simulink model "new_lv_try_control2"  (Simulink 7.1)
settings: Solver=ode3  StartTime=0.0  StopTime=150  FixedStep=0.01  RelTol=1e-3
values from neighbouring files (symbols this model uses):
  C = abs(d-B)    [fuzzycontrol.m]    (also in lv_demofile6.m = 1450000)
  Jem = 90    [lv_cankaofile.m]    (also in lv_demofile.m = 97.5; lv_demofile1.m = 97.5; lv_demofile2.m = 97.5; lv_demofile3.m = 97.5)
  Jwt = 9e7    (= 90000000)    [lv_cankaofile.m]    (also in lv_demofile.m = 3275300; lv_demofile1.m = 3275300; lv_demofile2.m = 3275300; lv_demofile3.m = 3275300)
  K = 83    [lv_cankaofile.m]    (also in lv_demofile.m; lv_demofile1.m = 75.76; lv_demofile2.m; lv_demofile3.m = 75.76)
  R = 40    [lv_cankaofile.m]    (also in lv_demofile.m = 38.5; lv_demofile1.m = 38.75; lv_demofile2.m = 38.5; lv_demofile3.m = 38.5)
  ro_air = 1.225    [lv_cankaofile.m]    (also in lv_demofile.m = 1.2236; lv_demofile1.m; lv_demofile2.m = 1.2236; lv_demofile3.m)
libraries: wt_blockset_v3 x2, simulink_extras x1, simulink x1, DRlib x1
settings Model: Creator=lv  LastModifiedBy=lv

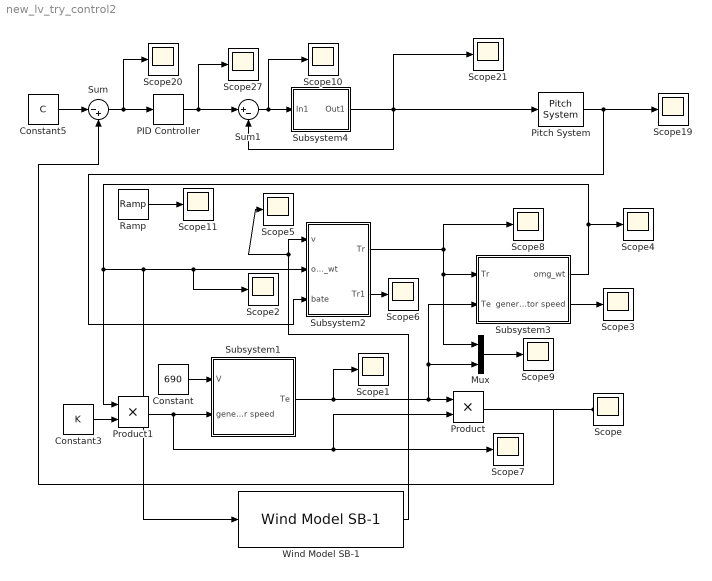
== system new_lv_try_control2 ==
  Constant : Constant  Value=690  OutDataType=sfix(16)  OutScaling=2^0
  Constant3 : Constant  Value=K  OutDataType=sfix(16)  OutScaling=2^0
  Constant5 : Constant  Value=C  OutDataType=sfix(16)  OutScaling=2^0
  Mux : Mux  Inputs=2
  PID Controller : simulink_extras/Additional Linear/PID Controller  SystemSampleTime=-1  P=15  I=0.002  D=1.1
  Pitch System : wt_blockset_v3/Control/WT Controller 2 MW DFIG/Pitch System  SystemSampleTime=-1
      link override Saturation1: LowerLimit=-90
  Product : Product  OutDataType=sfix(16)  OutScaling=2^0  RndMeth=Zero
  Product1 : Product  OutDataType=sfix(16)  OutScaling=2^0  RndMeth=Zero
  Ramp : simulink/Sources/Ramp  SystemSampleTime=-1  slope=-0.05  start=0  X0=16
  Scope{,1..11,19..21,27} (16 alike) : Scope
      Scope settings: TimeRange=100  YMin=700000  YMax=1.7e+006  SaveName=ScopeData9
      Scope1 settings: YMin=3424.13  YMax=3784.57  SaveName=ScopeData13
      Scope10 settings: YMin=-2.325e+007  YMax=-1.875e+007  SaveName=ScopeData28
      Scope11 settings: SaveName=ScopeData26
      Scope19 settings: YMin=27.2  YMax=27.285
      Scope2 settings: SaveName=ScopeData14
      Scope20 settings: YMin=-51201.2  YMax=-51201.1  SaveName=ScopeData11
      Scope21 settings: YMin=-2.325e+007  YMax=-1.875e+007  SaveName=ScopeData12
      Scope27 settings: YMin=-1.8e+007  YMax=-4e+006  SaveName=ScopeData27
      Scope3 settings: YMin=75.6077  YMax=83.5665  SaveName=ScopeData15
      Scope4 settings: YMin=1.96962  YMax=1.96971  SaveName=ScopeData16
      Scope5 settings: SaveName=ScopeData17
      Scope6 settings: SaveName=ScopeData18
      Scope7 settings: YMin=292.336  YMax=292.336  SaveName=ScopeData19
      Scope8 settings: YMin=725000  YMax=1.025e+006  SaveName=ScopeData22
      Scope9 settings: TimeRange=12  YMin=0  YMax=275000  SaveName=ScopeData2
  Subsystem1 : Subsystem
  Subsystem2 : Subsystem
  Subsystem3 : Subsystem
  Subsystem4 : Subsystem
  Sum : Sum  Inputs=|-+  OutDataType=sfix(16)  OutScaling=2^0  SaturateOnIntegerOverflow=on
  Sum1 : Sum  Inputs=|+-  OutDataType=sfix(16)  OutScaling=2^0  SaturateOnIntegerOverflow=on
  Wind Model SB-1 : wt_blockset_v3/Mechanical Components/Wind Model SB-1  SystemSampleTime=-1  D_rotor=77  v_mean=22  roughness=600  turb_int=12  T_sample=0.01
  wires:
  Subsystem1/1(Te) -> Product/1, Subsystem3/2(Te), Mux/2, Scope1/1
  Subsystem3/2(generator speed) -> Scope3/1
  Constant/1 -> Subsystem1/1(V)
  Subsystem3/1(omg_wt) -> Scope4/1, Product1/1, Subsystem2/2(omg_wt), Scope2/1, Wind Model SB-1/1
  Product/1 -> Scope/1, Sum/2
  Subsystem2/2(Tr1) -> Scope6/1
  Constant3/1 -> Product1/2
  Product1/1 -> Subsystem1/2(generator speed), Product/2, Scope7/1
  Subsystem2/1(Tr) -> Subsystem3/1(Tr), Mux/1, Scope8/1
  Mux/1 -> Scope9/1
  Sum/1 -> PID Controller/1, Scope20/1
  Constant5/1 -> Sum/1
  PID Controller/1 -> Scope27/1, Sum1/1
  Pitch System/1 -> Scope19/1, Subsystem2/3(bate)
  Subsystem4/1(Out1) -> Scope21/1, Sum1/2, Pitch System/1
  Sum1/1 -> Subsystem4/1(In1), Scope10/1
  Ramp/1 -> Scope11/1
  Wind Model SB-1/1 -> Scope5/1, Subsystem2/1(v)

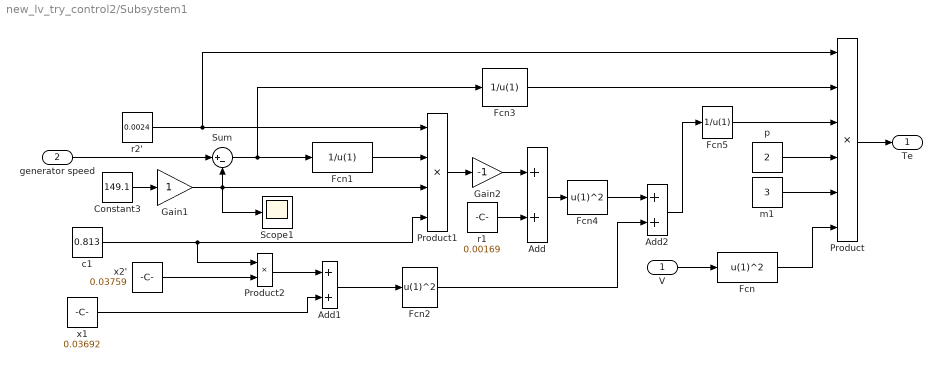
== system new_lv_try_control2/Subsystem1 ==
  V : Inport  OutDataType=sfix(16)  OutScaling=2^0
  generator speed : Inport  Port=2  OutDataType=sfix(16)  OutScaling=2^0
  Add : Sum  OutDataType=sfix(16)  OutScaling=2^-10
  Add1 : Sum  OutDataType=sfix(16)  OutScaling=2^-10
  Add2 : Sum  OutDataType=sfix(16)  OutScaling=2^-10
  Constant3 : Constant  Value=149.1  OutDataType=sfix(16)  OutScaling=2^0
  Fcn : Fcn  Expr=u(1)^2
  Fcn1 : Fcn  Expr=1/u(1)
  Fcn2 : Fcn  Expr=u(1)^2
  Fcn3 : Fcn  Expr=1/u(1)
  Fcn4 : Fcn  Expr=u(1)^2
  Fcn5 : Fcn  Expr=1/u(1)
  Gain1 : Gain  ParameterDataType=sfix(16)  ParameterScaling=2^0  OutDataType=sfix(16)  OutScaling=2^0
  Gain2 : Gain  Gain=-1  ParameterDataType=sfix(16)  ParameterScaling=2^0  OutDataType=sfix(16)  OutScaling=2^0
  Product : Product  Inputs=6  OutDataType=sfix(16)  OutScaling=2^0  RndMeth=Zero
  Product1 : Product  Inputs=4  OutDataType=sfix(16)  OutScaling=2^0  RndMeth=Zero
  Product2 : Product  OutDataType=sfix(16)  OutScaling=2^0  RndMeth=Zero
  Scope1 : Scope
      settings: SaveName=ScopeData10
  Sum : Sum  Inputs=|+-  OutDataType=sfix(16)  OutScaling=2^0
  c1 : Constant  Value=0.813  OutDataType=sfix(16)  OutScaling=2^0
  m1 : Constant  Value=3  OutDataType=sfix(16)  OutScaling=2^0
  p : Constant  Value=2  OutDataType=sfix(16)  OutScaling=2^0
  r1 : Constant  Value=0.00169  OutDataType=sfix(16)  OutScaling=2^0
  r2' : Constant  Value=0.0024  OutDataType=sfix(16)  OutScaling=2^0
  x1 : Constant  Value=0.03692  OutDataType=sfix(16)  OutScaling=2^0
  x2' : Constant  Value=0.03759  OutDataType=sfix(16)  OutScaling=2^0
  Te : Outport  OutDataType=sfix(16)  OutScaling=2^0
  wires:
  V/1 -> Fcn/1
  generator speed/1 -> Sum/1
  Constant3/1 -> Gain1/1
  Gain1/1 -> Sum/2, Product1/3, Scope1/1
  Sum/1 -> Fcn3/1, Fcn1/1
  r2'/1 -> Product1/1, Product/1
  Fcn1/1 -> Product1/2
  c1/1 -> Product1/4, Product2/1
  x2'/1 -> Product2/2
  Product2/1 -> Add1/1
  x1/1 -> Add1/2
  Add1/1 -> Fcn2/1
  Product1/1 -> Gain2/1
  r1/1 -> Add/2
  Gain2/1 -> Add/1
  Add/1 -> Fcn4/1
  Fcn4/1 -> Add2/1
  Fcn2/1 -> Add2/2
  Add2/1 -> Fcn5/1
  Product/1 -> Te/1
  Fcn3/1 -> Product/2
  Fcn5/1 -> Product/3
  p/1 -> Product/4
  m1/1 -> Product/5
  Fcn/1 -> Product/6

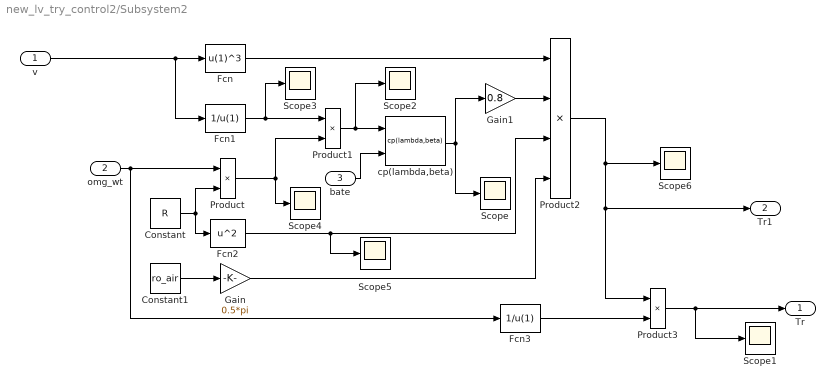
== system new_lv_try_control2/Subsystem2 ==
  v : Inport  OutDataType=sfix(16)  OutScaling=2^0
  omg_wt : Inport  Port=2  OutDataType=sfix(16)  OutScaling=2^0
  bate : Inport  Port=3  OutDataType=sfix(16)  OutScaling=2^0
  Constant : Constant  Value=R  OutDataType=sfix(16)  OutScaling=2^0
  Constant1 : Constant  Value=ro_air  OutDataType=sfix(16)  OutScaling=2^0
  Fcn : Fcn  Expr=u(1)^3
  Fcn1 : Fcn  Expr=1/u(1)
  Fcn2 : Fcn  Expr=u^2
  Fcn3 : Fcn  Expr=1/u(1)
  Gain : Gain  Gain=0.5*pi  ParameterDataType=sfix(16)  ParameterScaling=2^0  OutDataType=sfix(16)  OutScaling=2^0
  Gain1 : Gain  Gain=0.8  ParameterDataType=sfix(16)  ParameterScaling=2^0  OutDataType=sfix(16)  OutScaling=2^0
  Product : Product  OutDataType=sfix(16)  OutScaling=2^0  RndMeth=Zero
  Product1 : Product  OutDataType=sfix(16)  OutScaling=2^0  RndMeth=Zero
  Product2 : Product  Inputs=4  OutDataType=sfix(16)  OutScaling=2^0  RndMeth=Zero
  Product3 : Product  OutDataType=sfix(16)  OutScaling=2^0  RndMeth=Zero
  Scope{,1..6} (7 alike) : Scope
      Scope settings: TimeRange=50  YMin=0.1772981595092024  YMax=0.2028981595092024  SaveName=ScopeData4
      Scope1 settings: TimeRange=20  YMin=-1500000  YMax=1500000
      Scope2 settings: SaveName=ScopeData6
      Scope3 settings: SaveName=ScopeData7
      Scope4 settings: SaveName=ScopeData8
      Scope5 settings: YMin=1426.48  YMax=1576.64  SaveName=ScopeData20
      Scope6 settings: TimeRange=20  YMin=-500000  YMax=5e+006  SaveName=ScopeData21
  cp(lambda,beta) : DRlib/Wind Generation/Wind Turbine/cp(lambda,beta)  SystemSampleTime=-1
  Tr : Outport  OutDataType=sfix(16)  OutScaling=2^0
  Tr1 : Outport  Port=2  OutDataType=sfix(16)  OutScaling=2^0
  wires:
  v/1 -> Fcn/1, Fcn1/1
  omg_wt/1 -> Product/1, Fcn3/1
  Constant/1 -> Product/2, Fcn2/1
  Fcn1/1 -> Product1/1, Scope3/1
  Product/1 -> Product1/2, Scope4/1
  Product1/1 -> Scope2/1, cp(lambda,beta)/1
  bate/1 -> cp(lambda,beta)/2
  Fcn/1 -> Product2/1
  cp(lambda,beta)/1 -> Scope/1, Gain1/1
  Fcn2/1 -> Product2/3, Scope5/1
  Gain/1 -> Product2/4
  Constant1/1 -> Gain/1
  Product2/1 -> Scope6/1, Product3/1, Tr1/1
  Fcn3/1 -> Product3/2
  Product3/1 -> Scope1/1, Tr/1
  Gain1/1 -> Product2/2

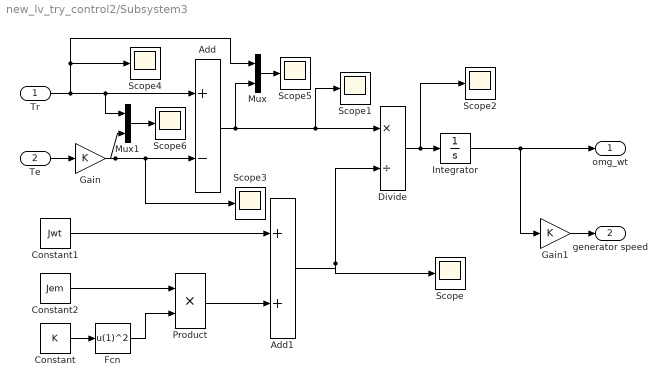
== system new_lv_try_control2/Subsystem3 ==
  Tr : Inport  OutDataType=sfix(16)  OutScaling=2^0
  Te : Inport  Port=2  OutDataType=sfix(16)  OutScaling=2^0
  Add : Sum  Inputs=+-  OutDataType=sfix(16)  OutScaling=2^-10
  Add1 : Sum  OutDataType=sfix(16)  OutScaling=2^-10
  Constant : Constant  Value=K  OutDataType=sfix(16)  OutScaling=2^0
  Constant1 : Constant  Value=Jwt  OutDataType=sfix(16)  OutScaling=2^0
  Constant2 : Constant  Value=Jem  OutDataType=sfix(16)  OutScaling=2^0
  Divide : Product  Inputs=*/  OutDataType=sfix(16)  OutScaling=2^-10
  Fcn : Fcn  Expr=u(1)^2
  Gain : Gain  Gain=K  ParameterDataType=sfix(16)  ParameterScaling=2^0  OutDataType=sfix(16)  OutScaling=2^0
  Gain1 : Gain  Gain=K  ParameterDataType=sfix(16)  ParameterScaling=2^0  OutDataType=sfix(16)  OutScaling=2^0
  Integrator : Integrator  InitialCondition=1.96885526
  Mux : Mux  Inputs=2
  Mux1 : Mux  Inputs=2
  Product : Product  OutDataType=sfix(16)  OutScaling=2^0  RndMeth=Zero
  Scope{,1..6} (7 alike) : Scope
      Scope settings: SaveName=ScopeData5
      Scope1 settings: YMin=1.3446e-008  YMax=1.3446e-008  SaveName=ScopeData6
      Scope2 settings: SaveName=ScopeData7
      Scope3 settings: SaveName=ScopeData23
      Scope4 settings: SaveName=ScopeData24
      Scope5 settings: SaveName=ScopeData25
      Scope6 settings: YMin=326577  YMax=326577  SaveName=ScopeData3
  omg_wt : Outport  OutDataType=sfix(16)  OutScaling=2^0
  generator speed : Outport  Port=2  OutDataType=sfix(16)  OutScaling=2^0
  wires:
  Fcn/1 -> Product/2
  Constant/1 -> Fcn/1
  Te/1 -> Gain/1
  Tr/1 -> Scope4/1, Mux/1, Add/1, Mux1/1
  Gain/1 -> Add/2, Scope3/1, Mux1/2
  Constant2/1 -> Product/1
  Constant1/1 -> Add1/1
  Product/1 -> Add1/2
  Add/1 -> Scope1/1, Divide/1, Mux/2
  Add1/1 -> Scope/1, Divide/2
  Divide/1 -> Scope2/1, Integrator/1
  Integrator/1 -> Gain1/1, omg_wt/1
  Gain1/1 -> generator speed/1
  Mux/1 -> Scope5/1
  Mux1/1 -> Scope6/1

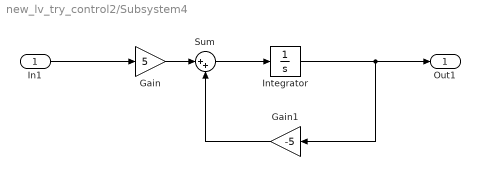
== system new_lv_try_control2/Subsystem4 ==
  In1 : Inport  OutDataType=sfix(16)  OutScaling=2^0
  Gain : Gain  Gain=5  ParameterDataType=sfix(16)  ParameterScaling=2^0  OutDataType=sfix(16)  OutScaling=2^0
  Gain1 : Gain  Orientation=left  Gain=-5  ParameterDataType=sfix(16)  ParameterScaling=2^0  OutDataType=sfix(16)  OutScaling=2^0
  Integrator : Integrator
  Sum : Sum  Inputs=|++  OutDataType=sfix(16)  OutScaling=2^0
  Out1 : Outport  OutDataType=sfix(16)  OutScaling=2^0
  wires:
  Integrator/1 -> Gain1/1, Out1/1
  Gain1/1 -> Sum/2
  Sum/1 -> Integrator/1
  Gain/1 -> Sum/1
  In1/1 -> Gain/1
